simulink model "Homing"  (R2024b)
settings: Solver=FixedStepAuto  StartTime=0.0  StopTime=30  FixedStep=0.01  RelTol=1e-3  EnableMultiTasking=on
libraries: stm32f4xxblockslib x1, stm32g4xxblockslib x1
settings Model: STM32="{\"AnalogInput\":{\"ID\":\"BasicKit:1\"},\"DigitalPortWrite\":{\"ID\":\"BasicKit:3\"},\"DigitalPortRead\":[{\"ID\":\"BasicKit:5\"},{\"ID\":\"BasicKit:7\"},{\"ID\":\"BasicKit:13\"},{\"ID\":\"BasicKit:14\"},{\"ID\":\"QEI:40\"},{\"ID\":\"QEI:41\"},{\"ID\":\"Read_Encoder:40\"},{\"ID\":\"Read_Encoder:41\"},{\"ID\":\"Homing:159\"}],\"EncoderBlockForG4\":[{\"ID\":\"BasicKit:9\"},{\"ID\":\"QEI:60\"},{\"ID\":\"QEI:61\"},{\"ID\":\"QEI:62\"},{\"ID\":\"Read_Encoder:62\"},{\"ID\":\"Read_Encoder:61\"},{\"ID\":\"Read_Encoder:60\"},{\"ID\":\"Homing:60\"}],\"HardwareInterrupt\":{\"ID\":\"Read_Encoder:142\"}}"  ExtModeBatchMode=on  Creator=beamk  LastModifiedBy=pboon
settings SolverCC: AutoInsertRateTranBlk=on
settings OptimizationCC: DefaultParameterBehavior=Inlined  EnhancedBackFolding=on  PassReuseOutputArgsAs=Individual arguments  ZeroExternalMemoryAtStartup=off  ZeroInternalMemoryAtStartup=off  MaxStackSize=512  OptimizeBlockOrder=speed  DifferentSizesBufferReuse=on  OptimizationCustomize=off  EfficientTunableParamExpr=on
settings DebuggingCC: ParameterTunabilityLossMsg=error
settings HardwareCC: ProdBitPerPointer=32  ProdBitPerSizeT=32  ProdBitPerPtrDiffT=32  ProdLargestAtomicInteger=Long  ProdLargestAtomicFloat=Double  ProdWordSize=32  ProdLongLongMode=on  ProdHWDeviceType=ARM Compatible->ARM Cortex-M
settings SFSimCC: MATLABDynamicMemAlloc=off
settings RTWCC: Description=Embedded Coder  SystemTargetFile=ert.tlc  HardwareBoard=STM32G4xx Based  TemplateMakefile=ert_default_tmf  Toolchain=GNU Tools for ARM Embedded Processors
settings CodeAppCC: ForceParamTrailComments=on  IgnoreCustomStorageClasses=off  OperatorAnnotations=on  SimulinkDataObjDesc=on  SFDataObjDesc=on  InsertBlockDesc=on
settings ERTTargetCC: TargetLangStandard=C99 (ISO)  CodeReplacementLibrary=ARM Cortex-M  SupportContinuousTime=on  ExtModeTransport=3  ExtModeStaticAlloc=on  ExtModeStaticAllocSize=2048  ExtModeMexFile=ext_xcp  ExtModeIntrfLevel=Level2 - Open

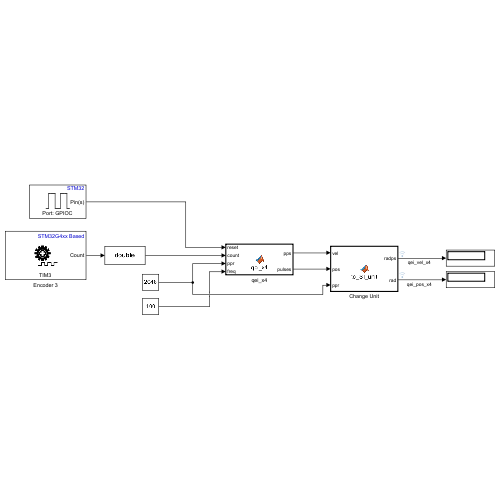
[thumbnail: Simulink's stored preview of the top-level diagram]
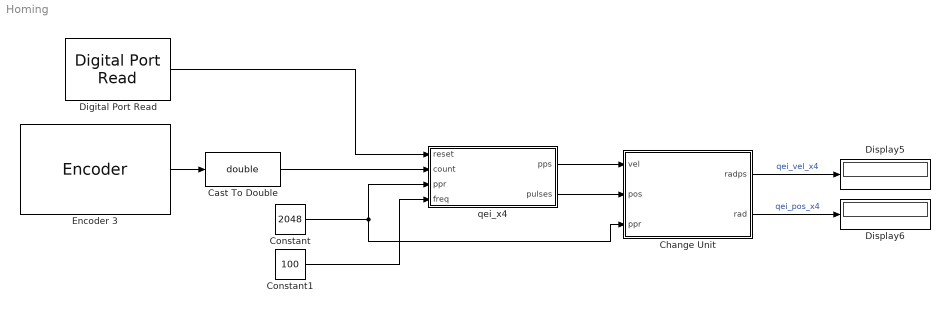
== system Homing ==
  Cast To Double : DataTypeConversion  OutDataTypeStr=double  SaturateOnIntegerOverflow=off  RndMeth=Floor
  Change Unit : MATLAB Function  TreatAsAtomicUnit=on
  Constant : Constant  Value=2048
  Constant1 : Constant  Value=100
  Digital Port Read : stm32f4xxblockslib/Digital Port Read  PortName=GPIOC  PinNumber=[13]  ReadOperation=on  IOAsArray=on  SampleTime=-1  EnableSimPort=off  hoistedMaskSrc=ECSoC/ECSimCodegen/Digital Port Read
      settings: LibrarySourceBlock=stm32g4xxblockslib/Digital Port Read
  Display5 : Display
  Display6 : Display
  Encoder 3 : stm32g4xxblockslib/Encoder  TimerModule=TIM3  EnableResetInput=off  OutputCountAfterFirstIndex=off  OutputValidIndex=off  OutputDirection=off  OutputStatus=off  SampleTime=-1
  qei_x4 : MATLAB Function  TreatAsAtomicUnit=on
  wires:
  Cast To Double/1 -> qei_x4/2(count)
  Encoder 3/1 -> Cast To Double/1
  qei_x4/1(pps) -> Change Unit/1(vel)
  qei_x4/2(pulses) -> Change Unit/2(pos)
  Change Unit/1(radps) -> Display5/1  "qei_vel_x4"
  Change Unit/2(rad) -> Display6/1  "qei_pos_x4"
  Constant/1 -> qei_x4/3(ppr), Change Unit/3(ppr)
  Constant1/1 -> qei_x4/4(freq)
  Digital Port Read/1 -> qei_x4/1(reset)

== matlab function Homing/qei_x4 ==
  data: reset input; count input; pps output; pulses output; ppr input; freq input
function [pps, pulses] = qei_x4(reset, count, ppr, freq)
enc_period = 65536 - mod(65536,ppr*4);
persistent prev_count
persistent pulses_accum
persistent diff_count

if isempty(prev_count)
    prev_count = 0;
end

if isempty(pulses_accum)
    pulses_accum = 0;
end

if isempty(diff_count)
    diff_count = 0;
end

if reset == 1
    pulses_accum = 0
end

diff_count = count - prev_count;

if diff_count > enc_period / 2
    diff_count = diff_count - enc_period;
elseif diff_count < -enc_period / 2
    diff_count = diff_count + enc_period;
end

pulses_accum = pulses_accum + diff_count;

pulses = pulses_accum;
pps = double(diff_count)*freq;

prev_count = count;
end

== matlab function Homing/Change Unit ==
  data: vel input; radps output; pos input; rad output; ppr input
function [radps, rad] = to_SI_unit(vel, pos, ppr)
    radps = (vel * 2 * pi) / ppr;

    rad = (pos * 2 * pi) / ppr;
end
